simulink model "res_filt"  (R2020a)
settings: Solver=VariableStepAuto  StartTime=0.0  StopTime=simulation.stopTime  RelTol=1e-3
undefined symbols (not defined in the file or in its folder): simulation
libraries: mcbcontrolslib x2
settings Model: Creator=FawadFarooq  LastModifiedBy=FawaD KhaN
settings DebuggingCC: SFMachineParentedDataDiag=error

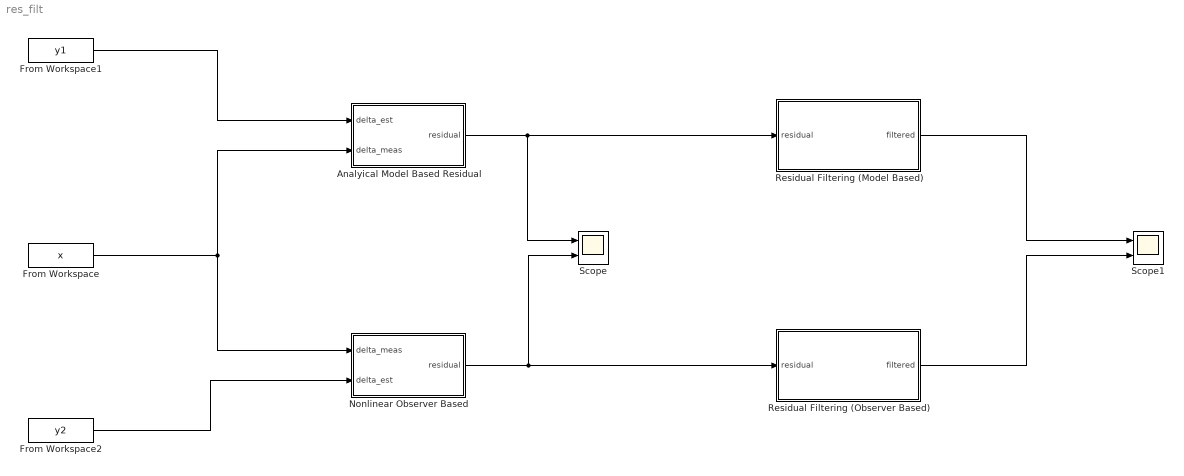
== system res_filt ==
  Analyical Model Based Residual : Subsystem
  From Workspace : FromWorkspace  VariableName=x  SampleTime=1/simulation.Fs
  From Workspace1 : FromWorkspace  VariableName=y1  SampleTime=1/simulation.Fs
  From Workspace2 : FromWorkspace  VariableName=y2  SampleTime=1/simulation.Fs
  Nonlinear Observer Based : Subsystem
  Residual Filtering (Model Based) : Subsystem
  Residual Filtering (Observer Based) : Subsystem
  Scope : Scope  NumInputPorts=2
  Scope1 : Scope  NumInputPorts=2
  wires:
  From Workspace/1 -> Analyical Model Based Residual/2(delta_meas), Nonlinear Observer Based/1(delta_meas)
  From Workspace1/1 -> Analyical Model Based Residual/1(delta_est)
  From Workspace2/1 -> Nonlinear Observer Based/2(delta_est)
  Analyical Model Based Residual/1(residual) -> Residual Filtering (Model Based)/1(residual), Scope/1
  Nonlinear Observer Based/1(residual) -> Residual Filtering (Observer Based)/1(residual), Scope/2
  Residual Filtering (Model Based)/1(filtered) -> Scope1/1
  Residual Filtering (Observer Based)/1(filtered) -> Scope1/2

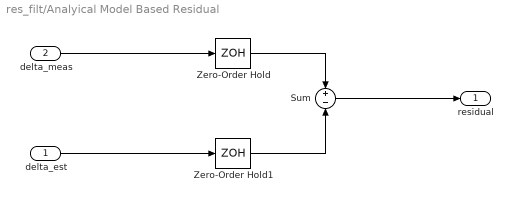
== system res_filt/Analyical Model Based Residual ==
  delta_est : Inport
  delta_meas : Inport  Port=2
  Sum : Sum  Inputs=+|-
  Zero-Order Hold : ZeroOrderHold  SampleTime=1/simulation.Fs
  Zero-Order Hold1 : ZeroOrderHold  SampleTime=1/simulation.Fs
  residual : Outport
  wires:
  Zero-Order Hold/1 -> Sum/1
  delta_meas/1 -> Zero-Order Hold/1
  delta_est/1 -> Zero-Order Hold1/1
  Zero-Order Hold1/1 -> Sum/2
  Sum/1 -> residual/1

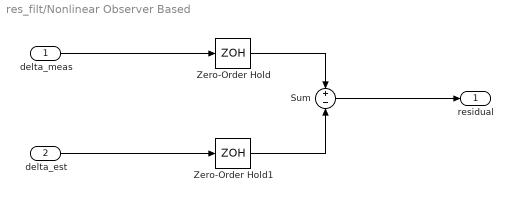
== system res_filt/Nonlinear Observer Based ==
  delta_meas : Inport
  delta_est : Inport  Port=2
  Sum : Sum  Inputs=+|-
  Zero-Order Hold : ZeroOrderHold  SampleTime=1/simulation.Fs
  Zero-Order Hold1 : ZeroOrderHold  SampleTime=1/simulation.Fs
  residual : Outport
  wires:
  Sum/1 -> residual/1
  Zero-Order Hold1/1 -> Sum/2
  delta_est/1 -> Zero-Order Hold1/1
  delta_meas/1 -> Zero-Order Hold/1
  Zero-Order Hold/1 -> Sum/1

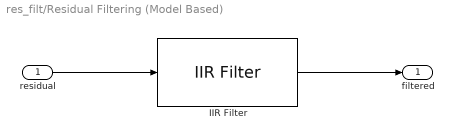
== system res_filt/Residual Filtering (Model Based) ==
  residual : Inport
  IIR Filter : mcbcontrolslib/IIR Filter  VariantControl=Low Pass Filter  Filter_constant=0.5
      settings: SourceProductBaseCode=MT
  filtered : Outport
  wires:
  IIR Filter/1 -> filtered/1
  residual/1 -> IIR Filter/1

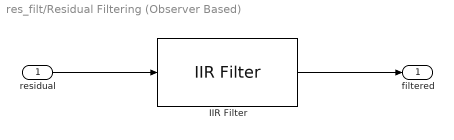
== system res_filt/Residual Filtering (Observer Based) ==
  residual : Inport
  IIR Filter : mcbcontrolslib/IIR Filter  VariantControl=Low Pass Filter  Filter_constant=0.5
      settings: SourceProductBaseCode=MT
  filtered : Outport
  wires:
  residual/1 -> IIR Filter/1
  IIR Filter/1 -> filtered/1
